simulink model "porsche_panamera_970_series_hybrid"  (R2024a)
settings: Solver=VariableStepAuto  StartTime=0.0  StopTime=1555  RelTol=1e-3
undefined symbols (not defined in the file or in its folder): eta_EM_map, H_u, P_aux, P_CE_cutoff, P_CE_idle, T_CE_cutoff, T_CE_max, T_EM_max, theta_CE, theta_EM, V_CE_map, w_CE_idle, w_CE_max, w_CE_upper, w_EM_row, w_EM_upper
libraries: qss_tb_library x7
settings Model: Creator=inser  LastModifiedBy=inser

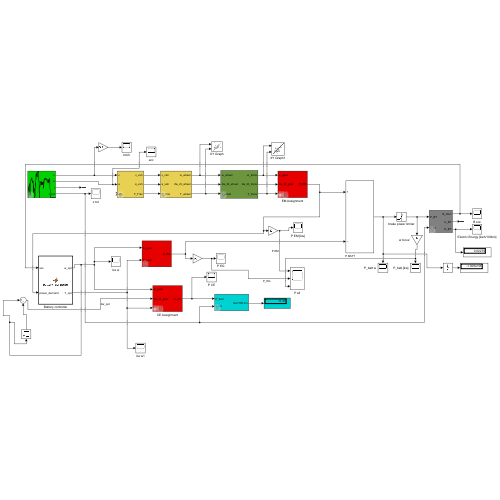
[thumbnail: Simulink's stored preview of the top-level diagram]
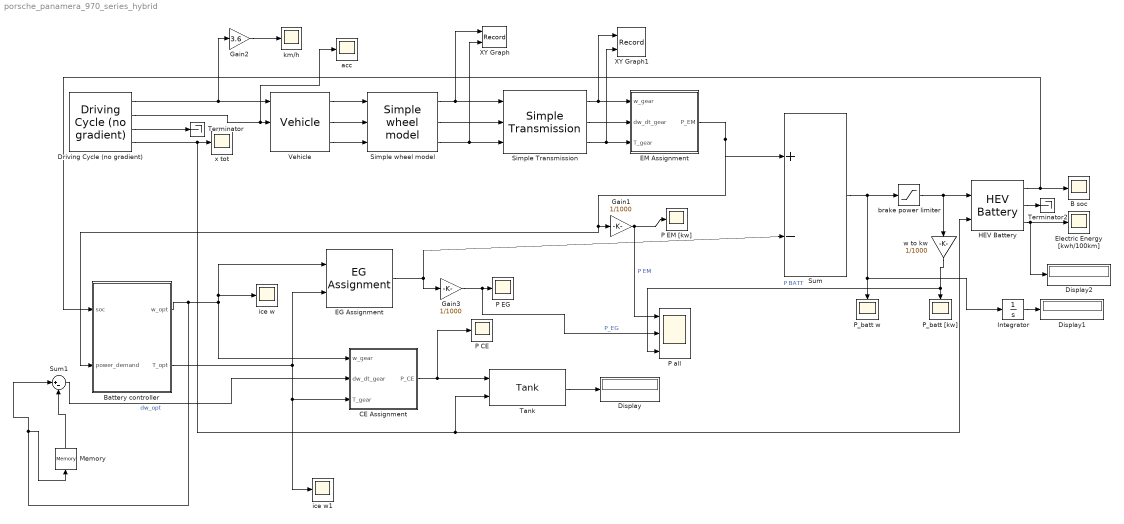
== system porsche_panamera_970_series_hybrid ==
  B soc : Scope
  Battery controller : MATLAB Function  TreatAsAtomicUnit=on
  CE Assignment : Subsystem  Tag=combustion engine  AncestorBlock=qss_tb_library/Energy Converter/CE Assignment  mask(Combustion Engine (based on consumption map)){engine_type=Gasoline, P_ice=300, ENABLE_FUEL_CUTOFF=on}
      mask prompts: engine_type "Engine type"; P_ice "Power [kW]"; ENABLE_FUEL_CUTOFF "Enable fuel cutoff"
      mask help:
      | This block simulates the behaviour of a combustion engine. The block is based on consumption maps for medium sized passenger cars.
      |
      | NA Gasoline:
      | max power @ 5000 rpm
      | max torque @ 3000 rpm
      |
      | Small Diesel:
      | max power @ 4500 rpm
      | max torque @ 2000 rpm
      |
      | Large Diesel:
      | max power @ 1500 rpm
      | max torque @ 1500 rpm
      |
      |
      | Input:
      | =====
      | 	w_gear	Speed of the fly wheel [rad/s]
      | 	dw_dt_gear	Acceleration of the fly wheel [rad/s^2]
      | 	T_gear	Torque on the fly wheel [Nm]
      |
      | Output:
      | ======
      | 	P_CE	Fuel power consumed by the combustion engine [W]
      mask init:
      | init_AssCE_map;
      mask TypeOptions engine_type: Gasoline | Small Diesel | Large Diesel
  Display : Display
  Display1 : Display
  Display2 : Display
  Driving Cycle (no gradient) : qss_tb_library/Driving Cycle/Driving Cycle (no gradient)  Tag=cycle  cyclename1=UD_DC_Porschev3  stepsize=1  autostop=on
  EG Assignment : qss_tb_library/Energy Converter/EG Assignment  P_eg=300
  EM Assignment : Subsystem  AncestorBlock=qss_tb_library/Energy Converter/EM Assignment  mask(Electric Motor){P_em=300}
      mask prompts: P_em "Power [kW]"
      mask help:
      | This block simulates the behaviour of an electric motor. The block is based on an efficiency map. The map is located in the Data/EnergyConvertter/ElectricMotor directory.
      |
      | Maximum speed och the electric motor is 6000 rpm
      | Field weakening region starts at 1500 rpm
      | Maximum mechanical power is at 2150 rpm
      | The maximum torque is 5.98 Nm/kW multiplied with the power you select.
      |
      | Input:
      | =====
      | 	w_gear	Speed of the motor [rad/s]
      | 	dw_dt_gear	Acceleration of the motor [rad/s^2]
      | 	T_gear	Torque of the motor [Nm]
      |
      | Output:
      | ======
      | 	P_EM	Electric Power consumed by the  motor [W]
      mask init:
      | init_EM_ass;
  Electric Energy [kwh/100km] : Scope
  Gain1 : Gain  Gain=1/1000
  Gain2 : Gain  Gain=3.6
  Gain3 : Gain  Gain=1/1000
  HEV Battery : qss_tb_library/Energy Buffer/HEV Battery  Tag=battery  cell_series=43  cell_parallel=1  Q_BT_IC_rel=39
  Integrator : Integrator
  Memory : Memory
  P CE : Scope
  P EG : Scope
  P EM [kw] : Scope
  P all : Scope  NumInputPorts=3
  P_batt [kw] : Scope
  P_batt w : Scope
  Simple Transmission : qss_tb_library/Gear System/Simple Transmission  Tag=simple transmission  gear_ratio=2  e_GT=0.98  P_GT0=50  w_wheel_min=1
  Simple wheel model : qss_tb_library/Vehicle/Simple wheel model  Tag=simple transmission  d_wheel=0.62
  Sum : Sum  Inputs=+|-
  Sum1 : Sum  Inputs=|+-
  Tank : qss_tb_library/Energy Source/Tank  Tag=tank  fuel=Gasoline  flag_cold_start=off
  Terminator : Terminator
  Terminator2 : Terminator
  Vehicle : qss_tb_library/Vehicle/Vehicle  Tag=vehicle  m_f=1731 + 200 + 150 + 100  A_f=2.3300  cw=0.3  mu=1.017/100  k_inertia=4
  XY Graph : Record  FileSettingsInternal="{\"entries\":[{\"content\":{\"excelSettings\":{\"content\":{},\"type\":\"Streamout.ExcelSettings\"}},\"type\":\"Streamout.FileSettingStorage\",\"uuid\":\"\"}],\"packageUris\":[\"http:\\/\\/schema.mathworks.com\\/mf0\\/streamout_blocks\\/R2020a\"],\"version\":\"1.0\"}"  Layout=[1 1]  SignalsInternal="{\"entries\":[{\"content\":{\"signals\":[{\"content\":{\"blockPath\":[],\"dimensions\":[1],\"domain\":\"\",\"lineColor\":\"#a2142f\",\"plots\":[ 1 ],\"port\":1,\"sid\":[\"\"],\"signalID\":1,\"signalName\":\"Simple wheel model:1\"},\"type\":\"RecordBlkView.Signal\",\"uuid\":\"\"},{\"content\":{\"blockPath\":[],\"dimensions\":[1],\"domain\":\"\",\"lineColor\":\"#139fff\",\"plots\":[ 1 ],\"port\":2,\"sid\":[\"\"],\"signalID\":2,\"signalName\":\"Simple wheel model:3\"},\"type\":\"RecordBlkView.Signal\",\"uuid\":\"\"}]},\"type\":\"RecordBlkView.InputSignals\",\"uuid\":\"\"}],\"packageUris\":[\"http:\\/\\/schema.mathworks.com\\/mf0\\/streamout_blocks\\/R2020a\"],\"version\":\"1.0\"}"  VisualizationBindings="{\"xyplotplugin\":{\"info\":[{\"series\":[{\"bindingParametersList\":[{\"parameter\":\"X-Axis\",\"signalID\":1,\"signalName\":\"Simple wheel model:1\"},{\"parameter\":\"Y-Axis\",\"signalID\":2,\"signalName\":\"Simple wheel model:3\"}],\"seriesID\":0}],\"subplotID\":1}]}}"  CompatibilityTag=XY
  XY Graph1 : Record  FileSettingsInternal="{\"entries\":[{\"content\":{\"excelSettings\":{\"content\":{},\"type\":\"Streamout.ExcelSettings\"}},\"type\":\"Streamout.FileSettingStorage\",\"uuid\":\"\"}],\"packageUris\":[\"http:\\/\\/schema.mathworks.com\\/mf0\\/streamout_blocks\\/R2020a\"],\"version\":\"1.0\"}"  Layout=[1 1]  SignalsInternal="{\"entries\":[{\"content\":{\"signals\":[{\"content\":{\"blockPath\":[],\"dimensions\":[1],\"domain\":\"\",\"lineColor\":\"#a2142f\",\"plots\":[ 1 ],\"port\":1,\"sid\":[\"\"],\"signalID\":1,\"signalName\":\"Simple Transmission:1\"},\"type\":\"RecordBlkView.Signal\",\"uuid\":\"\"},{\"content\":{\"blockPath\":[],\"dimensions\":[1],\"domain\":\"\",\"lineColor\":\"#139fff\",\"plots\":[ 1 ],\"port\":2,\"sid\":[\"\"],\"signalID\":2,\"signalName\":\"Simple Transmission:3\"},\"type\":\"RecordBlkView.Signal\",\"uuid\":\"\"}]},\"type\":\"RecordBlkView.InputSignals\",\"uuid\":\"\"}],\"packageUris\":[\"http:\\/\\/schema.mathworks.com\\/mf0\\/streamout_blocks\\/R2020a\"],\"version\":\"1.0\"}"  VisualizationBindings="{\"xyplotplugin\":{\"info\":[{\"series\":[{\"bindingParametersList\":[{\"parameter\":\"X-Axis\",\"signalID\":1,\"signalName\":\"Simple Transmission:1\"},{\"parameter\":\"Y-Axis\",\"signalID\":2,\"signalName\":\"Simple Transmission:3\"}],\"seriesID\":0}],\"subplotID\":1}]}}"  CompatibilityTag=XY
  acc : Scope
  brake power limiter : Saturate  UpperLimit=10e9  LowerLimit=-15*10^3
  ice w : Scope
  ice w1 : Scope
  km/h : Scope
  w to kw : Gain  Gain=1/1000
  x tot : Scope
  wires:
  Tank/1 -> Display/1
  Vehicle/3 -> Simple wheel model/3
  Vehicle/2 -> Simple wheel model/2
  Simple wheel model/1 -> Simple Transmission/1, XY Graph/1
  Simple wheel model/3 -> XY Graph/2, Simple Transmission/3
  Driving Cycle (no gradient)/1 -> Gain2/1, Vehicle/1
  Driving Cycle (no gradient)/2 -> acc/1, Vehicle/2
  Simple Transmission/1 -> XY Graph1/1, EM Assignment/1(w_gear)
  Simple Transmission/2 -> EM Assignment/2(dw_dt_gear)
  Simple Transmission/3 -> EM Assignment/3(T_gear), XY Graph1/2
  Vehicle/1 -> Simple wheel model/1
  Simple wheel model/2 -> Simple Transmission/2
  Driving Cycle (no gradient)/3 -> Terminator/1
  Sum/1 -> brake power limiter/1, Integrator/1, P_batt w/1
  Driving Cycle (no gradient)/4 -> HEV Battery/2, Tank/2, x tot/1
  CE Assignment/1(P_CE) -> P CE/1, Tank/1
  EG Assignment/1 -> Gain3/1, Sum/2
  HEV Battery/1 -> Battery controller/1(soc), B soc/1
  brake power limiter/1 -> HEV Battery/1, w to kw/1
  w to kw/1 -> P all/3, P_batt [kw]/1  "P BATT"
  HEV Battery/3 -> Electric Energy [kwh/100km]/1, Display2/1
  Battery controller/1(w_opt) -> Sum1/1, Memory/1, CE Assignment/1(w_gear), EG Assignment/1, ice w/1
  Battery controller/2(T_opt) -> CE Assignment/3(T_gear), ice w1/1, EG Assignment/2
  EM Assignment/1(P_EM) -> Battery controller/2(power_demand), Gain1/1, Sum/1
  Gain1/1 -> P all/1, P EM [kw]/1  "P EM"
  Integrator/1 -> Display1/1
  Gain2/1 -> km/h/1
  HEV Battery/2 -> Terminator2/1
  Gain3/1 -> P all/2, P EG/1  "P_EG"
  Memory/1 -> Sum1/2
  Sum1/1 -> CE Assignment/2(dw_dt_gear)  "dw_opt"

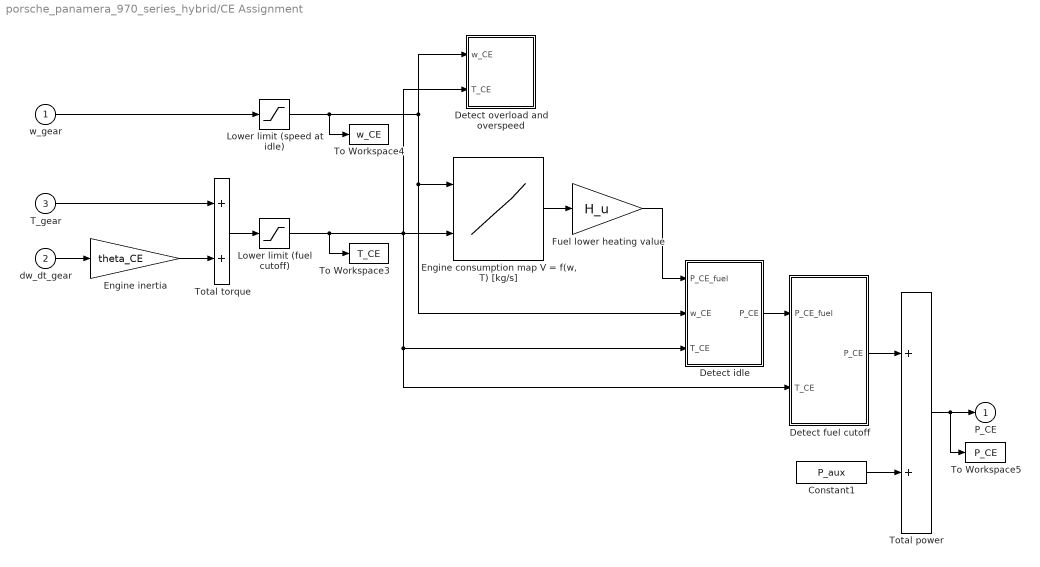
== system porsche_panamera_970_series_hybrid/CE Assignment ==
  w_gear : Inport
  dw_dt_gear : Inport  Port=2
  T_gear : Inport  Port=3
  Constant1 : Constant  Value=P_aux
  Detect fuel cutoff : Subsystem
  Detect idle : Subsystem
  Detect overload and overspeed : Subsystem
  "Engine consumption map V = f(w, T) [kg/s]" : Lookup2D  RowIndex=w_CE_row  ColumnIndex=T_CE_col  Table=V_CE_map  SaturateOnIntegerOverflow=off  InputSameDT=off
  Engine inertia : Gain  Gain=theta_CE  SaturateOnIntegerOverflow=on  OutDataTypeStr=Inherit: Same as input  ParamDataTypeStr=Inherit: Same as input
  Fuel lower heating value : Gain  Gain=H_u  SaturateOnIntegerOverflow=on  OutDataTypeStr=Inherit: Same as input  ParamDataTypeStr=Inherit: Same as input
  Lower limit (fuel cutoff) : Saturate  UpperLimit=inf  LowerLimit=T_CE_cutoff
  Lower limit (speed at idle) : Saturate  UpperLimit=inf  LowerLimit=w_CE_idle
  To Workspace3 : ToWorkspace  VariableName=T_CE  SampleTime=-1
  To Workspace4 : ToWorkspace  VariableName=w_CE  SampleTime=-1
  To Workspace5 : ToWorkspace  VariableName=P_CE  SampleTime=-1
  Total power : Sum  InputSameDT=on  SaturateOnIntegerOverflow=on  OutDataTypeStr=Inherit: Same as first input
  Total torque : Sum  InputSameDT=on  SaturateOnIntegerOverflow=on  OutDataTypeStr=Inherit: Same as first input
  P_CE : Outport  InitialOutput=0
  wires:
  T_gear/1 -> Total torque/1
  dw_dt_gear/1 -> Engine inertia/1
  Total torque/1 -> Lower limit (fuel cutoff)/1
  Engine inertia/1 -> Total torque/2
  Lower limit (speed at idle)/1 -> Detect overload and overspeed/1(w_CE), Detect idle/2(w_CE), "Engine consumption map V = f(w, T) [kg/s]"/1, To Workspace4/1
  w_gear/1 -> Lower limit (speed at idle)/1
  Fuel lower heating value/1 -> Detect idle/1(P_CE_fuel)
  Detect idle/1(P_CE) -> Detect fuel cutoff/1(P_CE_fuel)
  "Engine consumption map V = f(w, T) [kg/s]"/1 -> Fuel lower heating value/1
  Detect fuel cutoff/1(P_CE) -> Total power/1
  Total power/1 -> P_CE/1, To Workspace5/1
  Constant1/1 -> Total power/2
  Lower limit (fuel cutoff)/1 -> Detect overload and overspeed/2(T_CE), "Engine consumption map V = f(w, T) [kg/s]"/2, Detect idle/3(T_CE), Detect fuel cutoff/2(T_CE), To Workspace3/1

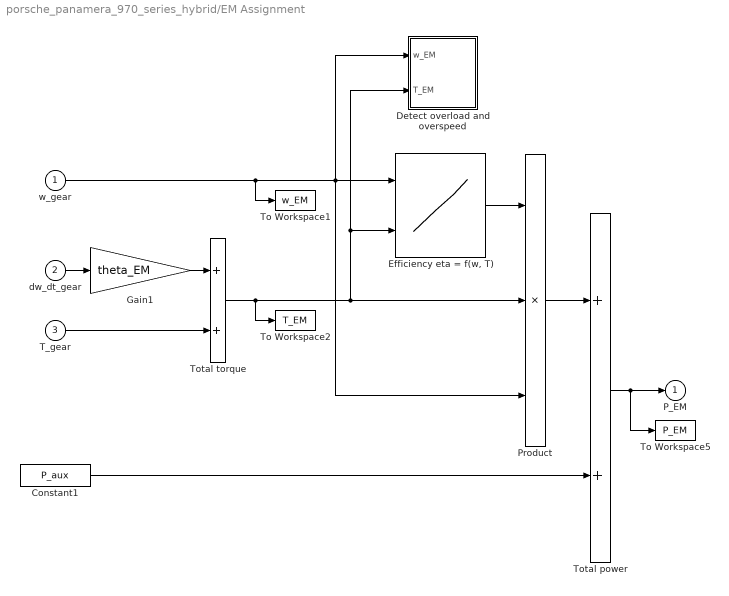
== system porsche_panamera_970_series_hybrid/EM Assignment ==
  w_gear : Inport
  dw_dt_gear : Inport  Port=2
  T_gear : Inport  Port=3
  Constant1 : Constant  Value=P_aux
  Detect overload and overspeed : Subsystem
  "Efficiency eta = f(w, T)" : Lookup2D  RowIndex=w_EM_row  ColumnIndex=T_EM_col  Table=eta_EM_map  SaturateOnIntegerOverflow=off  InputSameDT=off
  Gain1 : Gain  Gain=theta_EM  SaturateOnIntegerOverflow=on  OutDataTypeStr=Inherit: Same as input  ParamDataTypeStr=Inherit: Same as input
  Product : Product  Inputs=3  InputSameDT=on  RndMeth=Zero  SaturateOnIntegerOverflow=on  OutDataTypeStr=Inherit: Same as first input
  To Workspace1 : ToWorkspace  VariableName=w_EM  SampleTime=-1
  To Workspace2 : ToWorkspace  VariableName=T_EM  SampleTime=-1
  To Workspace5 : ToWorkspace  VariableName=P_EM  SampleTime=-1
  Total power : Sum  InputSameDT=on  SaturateOnIntegerOverflow=on  OutDataTypeStr=Inherit: Same as first input
  Total torque : Sum  InputSameDT=on  SaturateOnIntegerOverflow=on  OutDataTypeStr=Inherit: Same as first input
  P_EM : Outport  InitialOutput=0
  wires:
  Total power/1 -> To Workspace5/1, P_EM/1
  Product/1 -> Total power/1
  Constant1/1 -> Total power/2
  Total torque/1 -> To Workspace2/1, Product/2, "Efficiency eta = f(w, T)"/2, Detect overload and overspeed/2(T_EM)
  Gain1/1 -> Total torque/1
  T_gear/1 -> Total torque/2
  dw_dt_gear/1 -> Gain1/1
  "Efficiency eta = f(w, T)"/1 -> Product/1
  w_gear/1 -> To Workspace1/1, Product/3, "Efficiency eta = f(w, T)"/1, Detect overload and overspeed/1(w_EM)

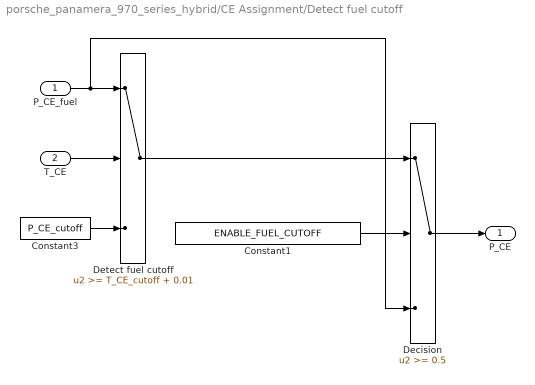
== system porsche_panamera_970_series_hybrid/CE Assignment/Detect fuel cutoff ==
  P_CE_fuel : Inport
  T_CE : Inport  Port=2
  Constant1 : Constant  Value=ENABLE_FUEL_CUTOFF
  Constant3 : Constant  Value=P_CE_cutoff
  Decision : Switch  Threshold=0.5  SaturateOnIntegerOverflow=off  InputSameDT=off
  Detect fuel cutoff : Switch  Threshold=T_CE_cutoff + 0.01
  P_CE : Outport
  wires:
  Constant3/1 -> Detect fuel cutoff/3
  T_CE/1 -> Detect fuel cutoff/2
  P_CE_fuel/1 -> Detect fuel cutoff/1, Decision/3
  Detect fuel cutoff/1 -> Decision/1
  Constant1/1 -> Decision/2
  Decision/1 -> P_CE/1

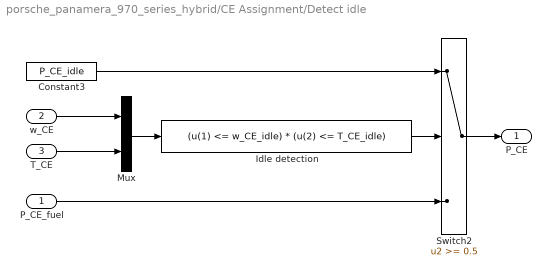
== system porsche_panamera_970_series_hybrid/CE Assignment/Detect idle ==
  P_CE_fuel : Inport
  w_CE : Inport  Port=2
  T_CE : Inport  Port=3
  Constant3 : Constant  Value=P_CE_idle
  Idle detection : Fcn  Expr=(u(1) <= w_CE_idle) * (u(2) <= T_CE_idle)
  Mux : Mux  Inputs=2
  Switch2 : Switch  Threshold=0.5
  P_CE : Outport  InitialOutput=0
  wires:
  Mux/1 -> Idle detection/1
  T_CE/1 -> Mux/2
  w_CE/1 -> Mux/1
  Idle detection/1 -> Switch2/2
  P_CE_fuel/1 -> Switch2/3
  Switch2/1 -> P_CE/1
  Constant3/1 -> Switch2/1

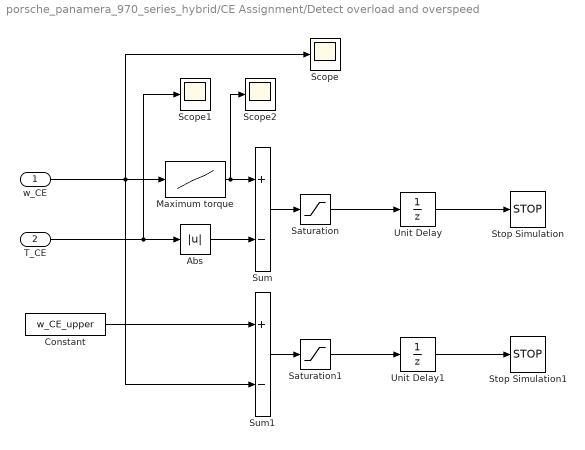
== system porsche_panamera_970_series_hybrid/CE Assignment/Detect overload and overspeed ==
  w_CE : Inport
  T_CE : Inport  Port=2
  Abs : Abs
  Constant : Constant  Value=w_CE_upper
  Maximum torque : Lookup  InputValues=w_CE_max  Table=T_CE_max
  Saturation : Saturate  UpperLimit=0  LowerLimit=-inf
  Saturation1 : Saturate  UpperLimit=0  LowerLimit=-inf
  Scope : Scope
  Scope1 : Scope
  Scope2 : Scope
  Stop Simulation : Stop
  Stop Simulation1 : Stop
  Sum : Sum  Inputs=+-  InputSameDT=on  SaturateOnIntegerOverflow=on  OutDataTypeStr=Inherit: Same as first input
  Sum1 : Sum  Inputs=+-  InputSameDT=on  SaturateOnIntegerOverflow=on  OutDataTypeStr=Inherit: Same as first input
  Unit Delay : UnitDelay  SampleTime=-1  HasFrameUpgradeWarning=on
  Unit Delay1 : UnitDelay  SampleTime=-1  HasFrameUpgradeWarning=on
  wires:
  Sum/1 -> Saturation/1
  w_CE/1 -> Maximum torque/1, Sum1/2, Scope/1
  T_CE/1 -> Abs/1, Scope1/1
  Maximum torque/1 -> Scope2/1, Sum/1
  Abs/1 -> Sum/2
  Saturation/1 -> Unit Delay/1
  Constant/1 -> Sum1/1
  Sum1/1 -> Saturation1/1
  Saturation1/1 -> Unit Delay1/1
  Unit Delay/1 -> Stop Simulation/1
  Unit Delay1/1 -> Stop Simulation1/1

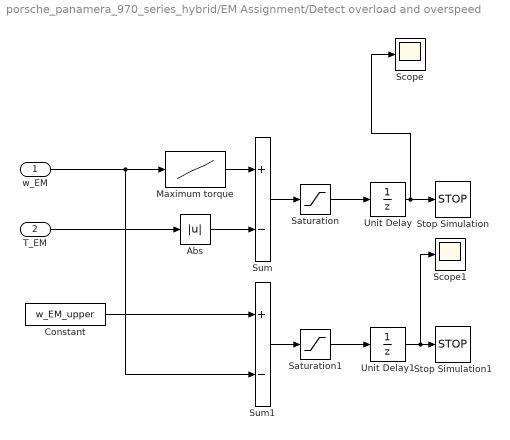
== system porsche_panamera_970_series_hybrid/EM Assignment/Detect overload and overspeed ==
  w_EM : Inport
  T_EM : Inport  Port=2
  Abs : Abs
  Constant : Constant  Value=w_EM_upper
  Maximum torque : Lookup  InputValues=w_EM_row  Table=T_EM_max
  Saturation : Saturate  UpperLimit=0  LowerLimit=-inf
  Saturation1 : Saturate  UpperLimit=0  LowerLimit=-inf
  Scope : Scope
  Scope1 : Scope
  Stop Simulation : Stop
  Stop Simulation1 : Stop
  Sum : Sum  Inputs=+-  InputSameDT=on  SaturateOnIntegerOverflow=on  OutDataTypeStr=Inherit: Same as first input
  Sum1 : Sum  Inputs=+-  InputSameDT=on  SaturateOnIntegerOverflow=on  OutDataTypeStr=Inherit: Same as first input
  Unit Delay : UnitDelay  SampleTime=-1  HasFrameUpgradeWarning=on
  Unit Delay1 : UnitDelay  SampleTime=-1  HasFrameUpgradeWarning=on
  wires:
  Sum/1 -> Saturation/1
  w_EM/1 -> Maximum torque/1, Sum1/2
  T_EM/1 -> Abs/1
  Maximum torque/1 -> Sum/1
  Abs/1 -> Sum/2
  Saturation/1 -> Unit Delay/1
  Constant/1 -> Sum1/1
  Sum1/1 -> Saturation1/1
  Saturation1/1 -> Unit Delay1/1
  Unit Delay/1 -> Scope/1, Stop Simulation/1
  Unit Delay1/1 -> Scope1/1, Stop Simulation1/1

== matlab function porsche_panamera_970_series_hybrid/Battery controller ==
  data: w_opt output; T_opt output; soc input; power_demand input
function [w_opt,T_opt] = battery_controller(soc, power_demand)
% Controller unit for battery in series hybrid
% Controlled by checking input power and SOC
% Group 15
 
% Input from fuel map
w = [1000,1380,2013,2456,2899,3342,3848,4500,4987,5177]; %[rpm]
T = [286,415,427,466,494,514,521,512,517,553]; % [Nm]

bsfc = [295,270,265,257,265,284,307,330,350,360] * (1/(3600e6)); %[kg/J]

% Define Power of ICE
power_ICE = 300; % Set ICE power [kw]
p_full = linspace(0,power_ICE,11);
p = p_full(2:end);

% Define the SOC limits
soc_min = 0.2;  % Battery start charge at 20%
soc_max = 0.9;  % Battery should stop charging at 90%


%------------------EFFICIENCY---------------------------%

% Good efficiency between 36 kw and 90 kw
power_ICE_high_eff_upper_limit = 209e3; 
power_ICE_best_eff = 120e3;              % Best operating point for ICE
power_ice_high_eff_lower_limit = 26e3;


LHV = 42.7e6; % [j/kg]
gen_efficiency = 0.9; % Assumed constant generator efficiency

power_demand_eff = 0; 

% ICE Power [W]
p_ice = (w * 2 * pi / 60) .* T;

% Fuel Power [W]
p_fuel = bsfc .* p_ice * LHV;

% ICE Efficiency
eta_ice = p_ice ./ p_fuel;

% Total Efficiency (ice + gen)
eta_total = eta_ice * gen_efficiency;

n_EGU = 0.8; % set fixed value for efficiency of EGU

%-----------------------CHARGING-------------------------------%

% Define persistent variable to track charging state
persistent charging;

if isempty(charging)
    charging = false; % Initially, assume the battery is not charging
end

% Define power limits based on power battery can provide
power_threshold = 9e3; % Power demand threshold [W]

% Initialize output variables
w_opt = 0;
T_opt = 0;


% ------------------ Charging Logig ------------------

if soc <= soc_min
    % If SOC is below 0.2 and power demand is low, start charging
    charging = true;  % Turn the charging switch ON
elseif soc >= soc_max 
    % If SOC is above 0.9 or power demand exceeds power threshhold, stop charging
    charging = false; % Turn the charging switch OFF    
end

% ------------------ Control logic based on charging state -------------------
if charging
    % Meet power demand + charge battery
    w_opt = interp1(p, w, ((power_demand/n_EGU) + power_threshold) / 1e3, 'linear', 'extrap') * 2 * pi / 60; % [rad/s] %
    T_opt = interp1(p, T, ((power_demand/n_EGU) + power_threshold) / 1e3, 'linear', 'extrap'); % [Nm]
    disp('charge')
    
    %Ensure that charging only happens until SOC reaches max value
    if soc >= soc_max 
        charging = false;  % Turn off charging once SOC is maxed out
        w_opt = 0;
        T_opt = 0;       
        disp('Turn of charging, Max soc!') 
  
    % Ensure battery cant discharge, charge to 30%
    elseif soc > 0.4 && power_demand < power_ice_high_eff_lower_limit
        charging = false;
        disp('Charging 30%')

    elseif soc >= 0.4 && power_demand >= power_ice_high_eff_lower_limit
        w_opt = interp1(p, w, ((power_demand/n_EGU) + power_threshold) / 1e3, 'linear', 'extrap') * 2 * pi / 60; % [rad/s] %
        T_opt = interp1(p, T, ((power_demand/n_EGU) + power_threshold) / 1e3, 'linear', 'extrap'); % [Nm]        
        disp('Charging 50%, power demand in efficient ICE region, charge more')
   
    end
    
elseif power_demand < 0 
    % Regenerative breaking, turn ICE OFF
    w_opt = 0;
    T_opt = 0;    
    disp('Regenerative breaking')

elseif power_demand >= 0 && power_demand < power_threshold % p <= 10
    % only use Battery Power for low power demands
    w_opt = 0;
    T_opt = 0;    
    disp('Only use battery')

elseif power_demand >= power_threshold 
    w_opt = interp1(p, w, ((power_demand/n_EGU) - power_threshold) / 1e3, 'linear', 'extrap') * 2 * pi / 60; % [rad/s]
    T_opt = interp1(p, T, ((power_demand/n_EGU) - power_threshold) / 1e3, 'linear', 'extrap'); % [Nm]   
    disp('Power demand exceed battery power, use battery and ICE, no charging')

    if power_demand >= (power_ICE_best_eff-30e3) && power_demand <= (power_ICE_best_eff+30e3) 
        w_opt = interp1(p, w, ((power_demand/n_EGU) + power_threshold) / 1e3, 'linear', 'extrap') * 2 * pi / 60; % [rad/s]
        T_opt = interp1(p, T, ((power_demand/n_EGU) + power_threshold) / 1e3, 'linear', 'extrap'); % [Nm]    
        disp('Power demand in efficient region, charge battery!')
    end
end
disp(power_demand/1e3)

% elseif power_demand >= power_ice_high_eff_lower_limit && power_demand <= power_ICE_high_eff_upper_limit
%     w_opt = interp1(p, w, ((power_demand/n_EGU) + power_threshold) / 1e3, 'linear', 'extrap') * 2 * pi / 60; % [rad/s]
%     T_opt = interp1(p, T, ((power_demand/n_EGU) + power_threshold) / 1e3, 'linear', 'extrap'); % [Nm]    
%     disp('Power demand in efficient region, charge battery!')
% 
% else
%     w_opt = interp1(p, w, ((power_demand/n_EGU) - power_threshold) / 1e3, 'linear', 'extrap') * 2 * pi / 60; % [rad/s]
%     T_opt = interp1(p, T, ((power_demand/n_EGU) - power_threshold) / 1e3, 'linear', 'extrap'); % [Nm]    
%     disp('Power demand in efficient region, charge battery!')



%-----------use above this-------------------------------------------------------------------------------------------------------------------------------



% elseif power_demand >= power_threshold && power_demand < power_ice_high_eff_lower_limit % 
%     % Just meet the power demand 
%     w_opt = interp1(p, w, ((power_demand/n_EGU) - power_threshold/n_EGU) / 1e3, 'linear', 'extrap') * 2 * pi / 60 % [rad/s]
%     T_opt = interp1(p, T, ((power_demand/n_EGU) - power_threshold/n_EGU) / 1e3, 'linear', 'extrap') % [Nm]
%     dw_opt = w_opt/5/n_EGU;
% 
%     % if soc >= soc_max
%     %     w_opt = interp1(p, w, power_demand/ 1e3, 'linear', 'extrap') * 2 * pi / 60 % [rad/s]
%     %     T_opt = interp1(p, T, power_demand / 1e3, 'linear', 'extrap') % [Nm]
%     % end
% 
% 
%     % w_opt = interp1(p, w, power_demand/ 1e3, 'linear', 'extrap') * 2 * pi / 60 % [rad/s]
%     % T_opt = interp1(p, T, power_demand / 1e3, 'linear', 'extrap') % [Nm]
%     % % 
%     disp('Meet power demand with ICE, low efficiency point of ICE, dont charge battery')
% 
% elseif power_demand >= power_ice_high_eff_lower_limit && power_demand < (power_ICE_best_eff - power_threshold) % 120-16 
%     % Just meet the power demand, near efficient point 
%     w_opt = interp1(p, w, (power_demand/n_EGU - power_threshold/n_EGU)/ 1e3, 'linear', 'extrap') * 2 * pi / 60 % [rad/s]
%     T_opt = interp1(p, T, (power_demand/n_EGU -power_threshold/n_EGU) / 1e3, 'linear', 'extrap') % [Nm]
%     dw_opt = w_opt/5/n_EGU;
%     disp('Within efficiency point, use battery')
% 
% 
% %--------------------- High power demand --------------------------------------------------------------------%    
% elseif power_demand >= (power_ICE_best_eff - power_threshold) && power_demand < power_ICE_best_eff %  p >= 56 and p <= 72
%     % Normal ICE operation at its best efficiency point also draw power
%     % from battery for optimal ICE operating point
%     w_opt = interp1(p, w, (power_demand/n_EGU - power_threshold/n_EGU) / 1e3, 'linear', 'extrap') * 2 * pi / 60; % [rad/s]
%     T_opt = interp1(p, T, (power_demand/n_EGU - power_threshold/n_EGU)  / 1e3, 'linear', 'extrap'); % [Nm]
%     dw_opt = w_opt/5/n_EGU;
%     disp('In most efficient region for operating')
% else
%     % Power demand is high
%     w_opt = interp1(p, w, (power_demand/n_EGU - power_threshold/n_EGU) / 1e3, 'linear', 'extrap') * 2 * pi / 60; % [rad/s]
%     T_opt = interp1(p, T, (power_demand/n_EGU - power_threshold/n_EGU) / 1e3, 'linear', 'extrap'); % [Nm]
%     dw_opt = w_opt/5/n_EGU;
%     disp('High power demand: Maximum power')
% 
% end    

















%%%%%%%%%%%%%%%%%%%%%%%%%%%%%%%%%%%%%%%%%%%%%%%%%%%%%%%%%%%%%%%%%%%%%%%%%%%%%%%%%%%%%%%%%%%%%%%%%%%%%%%%%%%%%%%%%%%%%%%%%%%%%%%%%%%%%%%%%%%%%%%%%%%%%
% 
% elseif power_demand >= (power_ICE_best_eff + power_threshold) && power_demand < ((power_ICE*10^3) - power_threshold) % p >= 72 + 16 = 88 and p < 164
%     % Power demand is higher than ICE power, no battery power
%     w_opt = interp1(p, w, power_demand / 1e3, 'linear', 'extrap') * 2 * pi / 60; % [rad/s]
%     T_opt = interp1(p, T, power_demand / 1e3, 'linear', 'extrap'); % [Nm]
%     disp('power_demand > (power_ICE_best_eff + power_threshold) % 72 + 16 = 88')
% 
% 
% elseif power_demand >= ((power_ICE*10^3) - power_threshold) % p >= 180 - 16 = 164
%     % High power demand, no charging or drawing power from battery
%     w_opt = (interp1(p, w, power_demand / 1e3, 'linear', 'extrap')) * 2 * pi / 60;  % Engine speed (rad/s)
%     T_opt = interp1(p, T, power_demand / 1e3, 'linear', 'extrap');  % Engine torque (Nm)
%     disp('power_demand >= ((power_ICE*10^3) - power_threshold) % p >= 180 - 16 = 164')



    
% 
%         % If charging is ON, charge the battery
% if charging && power_demand > power_threshold
%     w_opt = (interp1(p, w, (power_demand + power_threshold) / 1e3, 'linear', 'extrap')) * 2 * pi / 60;  % Engine speed (rad/s)
%     T_opt = interp1(p, T, (power_demand + power_threshold) / 1e3, 'linear', 'extrap');  % Engine torque (Nm)
%     %w_opt = (interp1(p, w, power_demand / 1e3, 'linear', 'extrap')) * 2 * pi / 60;  % Engine speed (rad/s)
%     %T_opt = interp1(p, T, power_demand / 1e3, 'linear', 'extrap');  % Engine torque (Nm)
% 
%     % For high powerdemand, dont charge
%     if power_demand >= (power_ICE-power_threshold)
%         w_opt = (interp1(p, w, power_demand / 1e3, 'linear', 'extrap')) * 2 * pi / 60;  % Engine speed (rad/s)
%         T_opt = interp1(p, T, power_demand / 1e3, 'linear', 'extrap');  % Engine torque (Nm)
%     end
% 
%     % Ensure that charging only happens until SOC reaches max value (0.7)
%     if soc >= soc_max
%         charging = false;  % Turn off charging once SOC is maxed out
%     end
% 
%     % Regenerative breaking, turn ICE OFF
% elseif power_demand < 0
%     w_opt = 0;
%     T_opt = 0;
% 
% else
%     % If charging is OFF, the battery can either supply power to the load
%     % or the system can run without the battery charge.
%     if power_demand >= power_ICE_best_eff && power_demand < (power_ICE_best_eff + power_threshold)            
%         % If power demand is high, provide power to EM, no charging
%         w_opt = (interp1(p, w, power_ICE_best_eff / 1e3, 'linear', 'extrap')) * 2 * pi / 60  % Engine speed (rad/s)
%         T_opt = interp1(p, T, power_ICE_best_eff / 1e3, 'linear', 'extrap')  % Engine torque (Nm)
% 
%     end
% end
% end


% if power_demand > 0
%         % Interpolation to get total efficiency at the requested power demand
%         tot_eff = interp1(p_ice, eta_total, power_demand, 'linear', 'extrap')
%     else
%         % If the power demand is zero or negative (e.g., regen), we don't need efficiency
%         tot_eff = 1; % Assumed efficiency during regeneration (100%)
% end
% 
% % Adjust Power Demand Based on Efficiency
% if power_demand > 0
%     power_demand_eff = power_demand / tot_eff % Adjusted demand
% else
%     power_demand_eff = power_demand % No adjustment for regeneration
% end
% 
% 
% % Battery high charged turn off ice
% if soc >= soc_max 
%     w_opt = 0;
%     T_opt = 0;
% 
% elseif soc < soc_min && power_demand > 0
%     w_opt = (interp1(p,w,power_demand/(1e3),"linear","extrap"))*2*pi/60;
%     T_opt = interp1(p,T,power_demand/(1e3),"linear","extrap");
% 
% % Battery low charged
% elseif soc <= 0.2 && power_demand > 0 
%     w_opt = (interp1(p,w,power_demand/(1e3),"linear","extrap"))*2*pi/60;
%     T_opt = interp1(p,T,power_demand/(1e3),"linear","extrap");
% 
% % Battery limit 16 kw, turn ice on if high power demand 
% elseif soc > 0.2 && power_demand >= 15e3
%     w_opt = (interp1(p,w,power_demand/(1e3),"linear","extrap"))*2*pi/60;
%     T_opt = interp1(p,T,power_demand/(1e3),"linear","extrap");
% 
% 
% 
% % Turn ice off for regen
% elseif soc > 0.2 && power_demand <= 0
%     w_opt = 0;
%     T_opt = 0;
% 
% % if low power demand, keep ice off
% elseif soc > 0.2 && soc < 0.9 && power_demand < 8e3
%     w_opt = 0; 
%     T_opt = 0;
% 
% elseif soc < 0.2
%     w_opt = (interp1(p,w,power_demand/(1e3),"linear","extrap"))*2*pi/60;
%     T_opt = interp1(p,T,power_demand/(1e3),"linear","extrap");
% end
% 
% 
% 
% end
%
